simulink model "tank_based_bi_teleop_pf_kalman"  (R2020b)
settings: Solver=FixedStepAuto  StartTime=0.0  StopTime=30  FixedStep=Ts  RelTol=1e-3
values from neighbouring files (symbols this model uses):
  A = 1    [four_channel_bilateral_teleoperation_kalman_params.m]    (also in four_channel_bilateral_teleoperation_params.m; kalman_test.m = [1 Ts Ts^2/2; 0 1 Ts; 0 0 1]; recursive_estimation.m = [1 Ts Ts^2/2; 0 1 Ts; 0 0 1]; scattering_based_bi_teleop_pf_kalman_params.m)
  alpha = 1    [tank_based_bi_teleop_pf_kalman.m]    (also in tank_based_bi_teleop_pf_params.m; tank_based_bi_teleop_pp_kalman.m; tank_based_bi_teleop_pp_params.m)
  Be = 100    [four_channel_bilateral_teleoperation_architecture_params.m]    (also in four_channel_bilateral_teleoperation_kalman_params.m = 0; four_channel_bilateral_teleoperation_params.m = 0; scattering_based_bi_teleop_pf_kalman_params.m = 10; scattering_based_bi_teleop_pf_params.m = 10)
  beta = 0.2    [tank_based_bi_teleop_pf_kalman.m]    (also in tank_based_bi_teleop_pf_params.m; tank_based_bi_teleop_pp_kalman.m; tank_based_bi_teleop_pp_params.m)
  Bh = 70    [four_channel_bilateral_teleoperation_architecture_params.m]    (also in four_channel_bilateral_teleoperation_kalman_params.m; four_channel_bilateral_teleoperation_params.m; scattering_based_bi_teleop_pf_kalman_params.m = 1.5; scattering_based_bi_teleop_pf_params.m = 1.5)
  Bs = 1    [four_channel_bilateral_teleoperation_architecture_params.m]    (also in four_channel_bilateral_teleoperation_kalman_params.m = 3.2; four_channel_bilateral_teleoperation_params.m = 3.2; scattering_based_bi_teleop_pf_kalman_params.m = 40; scattering_based_bi_teleop_pf_params.m = 3)
  delay = 1    [scattering_based_bi_teleop_pf_kalman_params.m]    (also in scattering_based_bi_teleop_pf_params.m; scattering_based_bi_teleop_pp_kalman_params.m; scattering_based_bi_teleop_pp_params.m; tank_based_bi_teleop_pf_kalman.m)
  Dm = 5    [four_channel_bilateral_teleoperation_architecture_params.m]    (also in four_channel_bilateral_teleoperation_kalman_params.m = 0; four_channel_bilateral_teleoperation_params.m = 0; scattering_based_bi_teleop_pf_kalman_params.m = 0; scattering_based_bi_teleop_pf_params.m = 0)
  Ds = 10    [four_channel_bilateral_teleoperation_architecture_params.m]    (also in four_channel_bilateral_teleoperation_kalman_params.m = 0; four_channel_bilateral_teleoperation_params.m = 0; scattering_based_bi_teleop_pf_kalman_params.m = 0; scattering_based_bi_teleop_pf_params.m = 0)
  Fc = 1    [four_channel_bilateral_teleoperation_kalman_params.m]    (also in four_channel_bilateral_teleoperation_params.m; kalman_test.m = 10; scattering_based_bi_teleop_pf_kalman_params.m = 0.1; scattering_based_bi_teleop_pf_params.m)
  Fip = 1    [four_channel_bilateral_teleoperation_kalman_params.m]    (also in four_channel_bilateral_teleoperation_params.m; scattering_based_bi_teleop_pf_kalman_params.m = 5; scattering_based_bi_teleop_pf_params.m; scattering_based_bi_teleop_pp_kalman_params.m = 5)
  h_limit = 1    [tank_based_bi_teleop_pf_kalman.m]    (also in tank_based_bi_teleop_pf_params.m; tank_based_bi_teleop_pp_kalman.m; tank_based_bi_teleop_pp_params.m = 1.5)
  H_master_init = 100    [tank_based_bi_teleop_pf_kalman.m]    (also in tank_based_bi_teleop_pf_params.m; tank_based_bi_teleop_pp_kalman.m = 5; tank_based_bi_teleop_pp_params.m = 1)
  H_slave_init = 100    [tank_based_bi_teleop_pf_kalman.m]    (also in tank_based_bi_teleop_pf_params.m; tank_based_bi_teleop_pp_kalman.m = 5; tank_based_bi_teleop_pp_params.m = 1)
  Ih = 2    [scattering_based_bi_teleop_pf_kalman_params.m]    (also in scattering_based_bi_teleop_pp_kalman_params.m; scattering_based_bi_teleop_pp_params.m; tank_based_bi_teleop_pf_kalman.m; tank_based_bi_teleop_pf_params.m)
  Je = 0    [four_channel_bilateral_teleoperation_architecture_params.m]    (also in four_channel_bilateral_teleoperation_kalman_params.m; four_channel_bilateral_teleoperation_params.m; scattering_based_bi_teleop_pf_kalman_params.m; scattering_based_bi_teleop_pf_params.m)
  Jh = 0.5    [four_channel_bilateral_teleoperation_architecture_params.m]    (also in four_channel_bilateral_teleoperation_kalman_params.m; four_channel_bilateral_teleoperation_params.m; scattering_based_bi_teleop_pf_kalman_params.m = 0; scattering_based_bi_teleop_pf_params.m = 0.05)
  Ke = 200    [four_channel_bilateral_teleoperation_architecture_params.m]    (also in four_channel_bilateral_teleoperation_kalman_params.m = 50; four_channel_bilateral_teleoperation_params.m = 50; scattering_based_bi_teleop_pf_kalman_params.m; scattering_based_bi_teleop_pf_params.m)
  Kh = 2000    [four_channel_bilateral_teleoperation_architecture_params.m]    (also in four_channel_bilateral_teleoperation_kalman_params.m; four_channel_bilateral_teleoperation_params.m; scattering_based_bi_teleop_pf_kalman_params.m = 1; scattering_based_bi_teleop_pf_params.m = 0)
  Ks = 1    [four_channel_bilateral_teleoperation_architecture_params.m]    (also in four_channel_bilateral_teleoperation_kalman_params.m = 4; four_channel_bilateral_teleoperation_params.m = 4; scattering_based_bi_teleop_pf_kalman_params.m = 50; scattering_based_bi_teleop_pf_params.m = 110)
  Mm = 0.5    [four_channel_bilateral_teleoperation_architecture_params.m]    (also in four_channel_bilateral_teleoperation_kalman_params.m; four_channel_bilateral_teleoperation_params.m; scattering_based_bi_teleop_pf_kalman_params.m; scattering_based_bi_teleop_pf_params.m)
  Ms = 2    [four_channel_bilateral_teleoperation_architecture_params.m]    (also in four_channel_bilateral_teleoperation_kalman_params.m; four_channel_bilateral_teleoperation_params.m; scattering_based_bi_teleop_pf_kalman_params.m; scattering_based_bi_teleop_pf_params.m)
  Ph = 2000    [four_channel_bilateral_teleoperation_kalman_params.m]    (also in four_channel_bilateral_teleoperation_params.m = 50500; scattering_based_bi_teleop_pf_kalman_params.m = 5; scattering_based_bi_teleop_pf_params.m = 23; scattering_based_bi_teleop_pp_kalman_params.m = 6)
  Ts = 0.001    [four_channel_bilateral_teleoperation_kalman_params.m]    (also in four_channel_bilateral_teleoperation_params.m; kalman_test.m; recursive_estimation.m; scattering_based_bi_teleop_pf_kalman_params.m)
  VarianceForces = 0.01    [four_channel_bilateral_teleoperation_kalman_params.m]    (also in four_channel_bilateral_teleoperation_params.m; scattering_based_bi_teleop_pf_kalman_params.m; scattering_based_bi_teleop_pp_kalman_params.m; scattering_based_bi_teleop_pp_params.m)
  VarianceVelocities = 0.001    [four_channel_bilateral_teleoperation_kalman_params.m]    (also in four_channel_bilateral_teleoperation_params.m; scattering_based_bi_teleop_pf_kalman_params.m = 1e-05; scattering_based_bi_teleop_pp_kalman_params.m = 1e-05; scattering_based_bi_teleop_pp_params.m = 1e-05)
settings Model: Creator=anuj  LastModifiedBy=filippo

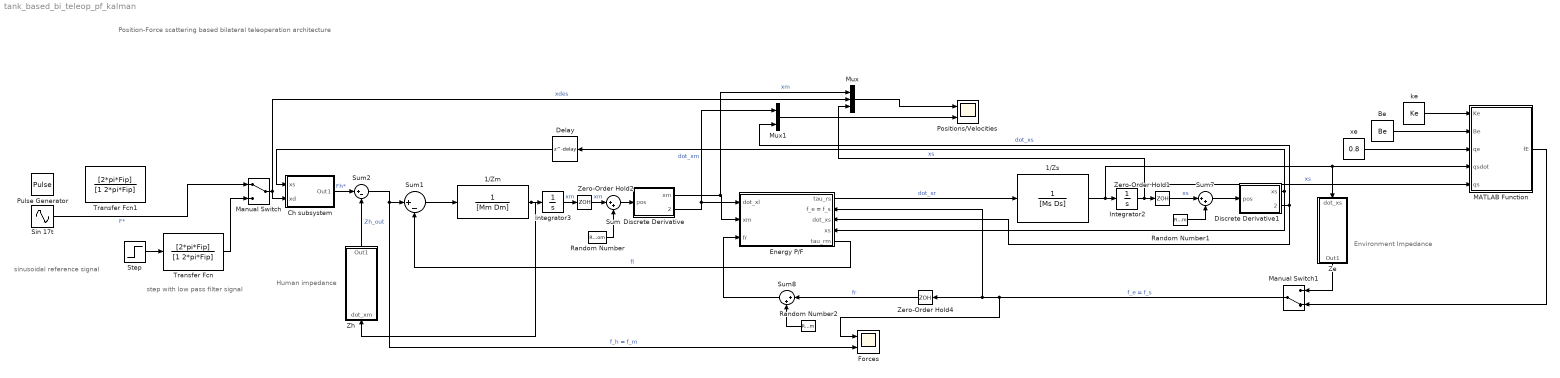
== system tank_based_bi_teleop_pf_kalman ==
  note: Position-Force scattering based bilateral teleoperation architecture
  note: Environment Impedance
  note: Human impedance
  note: sinusoidal reference signal
  note: step with low pass filter signal
  1/Zm : TransferFcn  Denominator=[Mm Dm]
  1/Zs : TransferFcn  Denominator=[Ms Ds]
  Be : Constant  Value=Be
  Ch subsystem : Subsystem
  Delay : Delay  DelayLength=delay  SampleTime=Ts
  Discrete Derivative : Subsystem
  Discrete Derivative1 : Subsystem
  Energy P/F : Subsystem
      settings: PortSchema="{\"entries\":[{\"content\":{\"sides\":[{\"content\":{\"connectorIds\":[\"In1\",\"In2\",\"In3\"]},\"type\":\"ConnectorPlacement.EquallySpacedRectSide\",\"uuid\":\"f2b5b233-4bc9-48fa-8c02-3c8bfabc8edf\"},{\"content\":{\"connectorIds\":[\"Out1\",\"In4\",\"In5\",\"In6\",\"Out2\"],\"side\":\"RIGHT\"},\"type\":\"ConnectorPlacement.EquallySpacedRectSide\",\"uuid\":\"567bdcc6-c695-4210-9521-fb074471be82\"},{\"content\":{\"connectorIds\":[],\"side\":\"TOP\"},\"type\":\"ConnectorPlacement.EquallySpacedRectSide\",\"uuid\":\"1a36b9db-f8a2-44fb-9901-095b7ca2258a\"},{\"content\":{\"connectorIds\":[],\"side\":\"HIDDEN\"},\"type\":\"ConnectorPlacement.EquallySpacedRectSide\",\"uuid\":\"2e8b54c5-18c4-4c1b-a8a4-ee42e67d82c7\"}]},\"type\":\"ConnectorPlacement.EquallySpacedConnector\",\"uuid\":\"569d959e-ea5b-42c6-b188-2deb8683cad8\"}],\"packageUris\":[\"http://schema.mathworks.com/mf0/Connector/R2020b\"],\"version\":\"1.0\"}"
  Forces : Scope  NumInputPorts=2
  Integrator2 : Integrator
  Integrator3 : Integrator
  MATLAB Function : MATLAB Function  TreatAsAtomicUnit=on
  Manual Switch : ManualSwitch
  Manual Switch1 : ManualSwitch  CurrentSetting=0
  Mux : Mux  Inputs=3
  Mux1 : Mux  Inputs=2
  Positions/Velocities : Scope  NumInputPorts=2
  Pulse Generator : DiscretePulseGenerator  PulseType=Time based  Amplitude=A  PulseWidth=50  PhaseDelay=1
  Random Number : RandomNumber  Variance=VarianceVelocities  SampleTime=Ts
  Random Number1 : RandomNumber  Variance=VarianceVelocities  SampleTime=Ts
  Random Number2 : RandomNumber  Variance=VarianceForces  SampleTime=Ts
  Sin 17t : Sin  Amplitude=A  Frequency=2*pi*Fc  SampleTime=0
  Step : Step  After=A  SampleTime=0
  Sum : Sum  Inputs=|++
  Sum1 : Sum  Inputs=|+-
  Sum2 : Sum  Inputs=|+-
  Sum7 : Sum  Inputs=|++
  Sum8 : Sum  Inputs=|++
  Transfer Fcn : TransferFcn  Numerator=[2*pi*Fip]  Denominator=[1 2*pi*Fip]
  Transfer Fcn1 : TransferFcn  Numerator=[2*pi*Fip]  Denominator=[1 2*pi*Fip]
  Ze : Subsystem
  Zero-Order Hold1 : ZeroOrderHold  SampleTime=Ts
  Zero-Order Hold2 : ZeroOrderHold  SampleTime=Ts
  Zero-Order Hold4 : ZeroOrderHold  SampleTime=Ts
  Zh : Subsystem
  ke : Constant  Value=Ke
  xe : Constant  Value=0.8
  wires:
  Sum2/1 -> Forces/2, Sum1/1  "f_h = f_m"
  1/Zm/1 -> Zh/1(dot_xm), Integrator3/1
  Sum1/1 -> 1/Zm/1
  Energy P/F/2(tau_rm) -> Sum1/2  "fl"
  Manual Switch1/1 -> Energy P/F/4(f_e = f_s), Zero-Order Hold4/1, Forces/1  "f_e = f_s"
  Be/1 -> MATLAB Function/2(Be)
  xe/1 -> MATLAB Function/3(qe)
  ke/1 -> MATLAB Function/1(Ke)
  Transfer Fcn/1 -> Manual Switch/2
  Step/1 -> Transfer Fcn/1
  Zh/1(Out1) -> Sum2/2  "Zh_out"
  Discrete Derivative1/2(dot_xs) -> Energy P/F/5(dot_xs), Mux1/2  "dot_xs"
  1/Zs/1 -> Integrator2/1, Ze/1(dot_xs), MATLAB Function/4(qsdot)
  Integrator2/1 -> Zero-Order Hold1/1, Mux/3, MATLAB Function/5(qs)  "xs"
  Zero-Order Hold1/1 -> Sum7/1  "xs"
  Integrator3/1 -> Zero-Order Hold2/1  "xm"
  Discrete Derivative/2(dot_xm) -> Mux1/1, Energy P/F/1(dot_xl)  "dot_xm"
  Ze/1(Out1) -> Manual Switch1/1
  MATLAB Function/1(fE) -> Manual Switch1/2
  Mux1/1 -> Positions/Velocities/2
  Mux/1 -> Positions/Velocities/1
  Manual Switch/1 -> Mux/2, Ch subsystem/2(xd)  "xdes"
  Ch subsystem/1(Out1) -> Sum2/1  "Fh*"
  Energy P/F/1(tau_rs) -> 1/Zs/1  "dot_xr"
  Delay/1 -> Ch subsystem/1(xs)
  Sin 17t/1 -> Manual Switch/1  "F*"
  Sum/1 -> Discrete Derivative/1(pos)
  Random Number/1 -> Sum/2
  Zero-Order Hold2/1 -> Sum/1  "xm"
  Discrete Derivative/1(xm) -> Mux/1, Energy P/F/2(xm)  "xm"
  Random Number2/1 -> Sum8/2
  Zero-Order Hold4/1 -> Sum8/1  "fr"
  Sum8/1 -> Energy P/F/3(fr)
  Random Number1/1 -> Sum7/2
  Sum7/1 -> Discrete Derivative1/1(pos)
  Discrete Derivative1/1(xs) -> Energy P/F/6(xs), Delay/1  "xs"

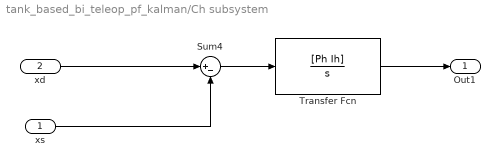
== system tank_based_bi_teleop_pf_kalman/Ch subsystem ==
  xs : Inport
  xd : Inport  Port=2
  Sum4 : Sum  Inputs=|+-
  Transfer Fcn : TransferFcn  Numerator=[Ph Ih]  Denominator=[1 0]
  Out1 : Outport
  wires:
  xd/1 -> Sum4/1
  xs/1 -> Sum4/2
  Sum4/1 -> Transfer Fcn/1
  Transfer Fcn/1 -> Out1/1

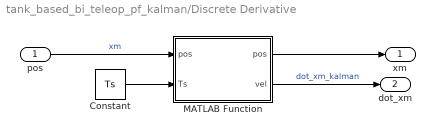
== system tank_based_bi_teleop_pf_kalman/Discrete Derivative ==
  pos : Inport
  Constant : Constant  Value=Ts
  MATLAB Function : MATLAB Function  TreatAsAtomicUnit=on
  xm : Outport
  dot_xm : Outport  Port=2
  wires:
  pos/1 -> MATLAB Function/1("pos ")  "xm"
  Constant/1 -> MATLAB Function/2(Ts)
  MATLAB Function/1(pos) -> xm/1
  MATLAB Function/2(vel) -> dot_xm/1  "dot_xm_kalman"

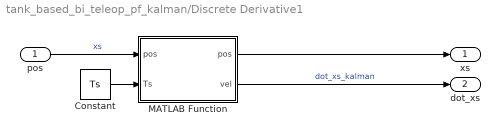
== system tank_based_bi_teleop_pf_kalman/Discrete Derivative1 ==
  pos : Inport
  Constant : Constant  Value=Ts
  MATLAB Function : MATLAB Function  TreatAsAtomicUnit=on
  xs : Outport
  dot_xs : Outport  Port=2
  wires:
  pos/1 -> MATLAB Function/1("pos ")  "xs"
  Constant/1 -> MATLAB Function/2(Ts)
  MATLAB Function/1(pos) -> xs/1
  MATLAB Function/2(vel) -> dot_xs/1  "dot_xs_kalman"

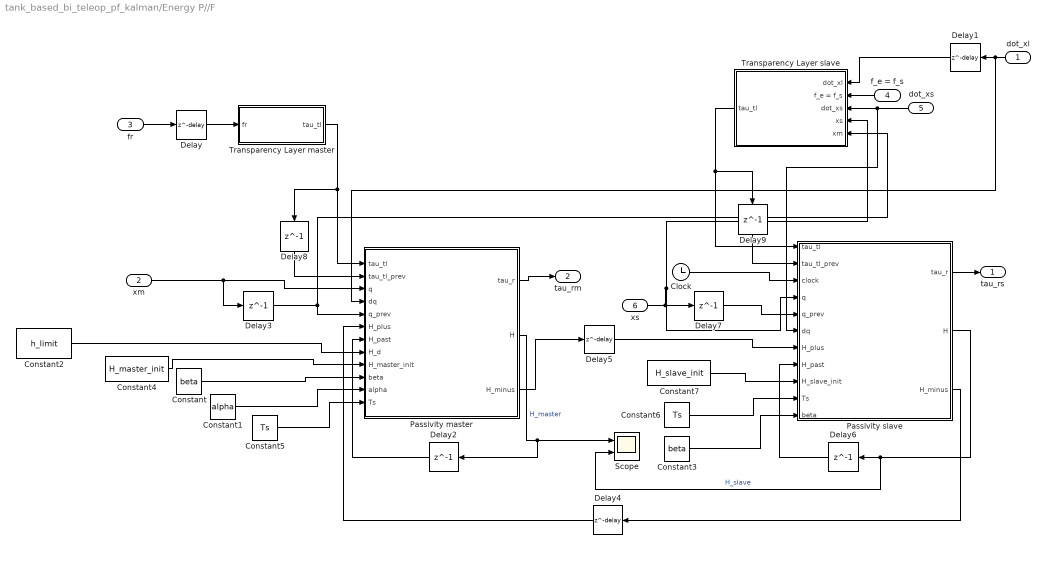
== system tank_based_bi_teleop_pf_kalman/Energy P//F ==
  dot_xl : Inport
  xm : Inport  Port=2
  fr : Inport  Port=3
  f_e = f_s : Inport  Port=4
  dot_xs : Inport  Port=5
  xs : Inport  Port=6
  Clock : Clock
  Constant : Constant  Value=beta
  Constant1 : Constant  Value=alpha
  Constant2 : Constant  Value=h_limit
  Constant3 : Constant  Value=beta
  Constant4 : Constant  Value=H_master_init
  Constant5 : Constant  Value=Ts
  Constant6 : Constant  Value=Ts
  Constant7 : Constant  Value=H_slave_init
  Delay{,1,4..5} (4 alike) : Delay  DelayLength=delay  SampleTime=Ts
  Delay{2..3,6..9} (6 alike) : Delay  DelayLength=1  SampleTime=Ts
  Passivity master : MATLAB Function  TreatAsAtomicUnit=on
  Passivity slave : MATLAB Function  TreatAsAtomicUnit=on
  Scope : Scope  NumInputPorts=2
  Transparency Layer master : Subsystem
  Transparency Layer slave : Subsystem
  tau_rs : Outport
  tau_rm : Outport  Port=2
  wires:
  dot_xl/1 -> Passivity master/4(dq), Delay1/1
  fr/1 -> Delay/1
  Delay2/1 -> Passivity master/7(H_past)
  xm/1 -> Passivity master/3(q), Delay3/1
  Delay3/1 -> Transparency Layer slave/5(xm), Passivity master/5(q_prev)
  Passivity slave/2(H) -> Scope/2, Delay6/1  "H_slave"
  Delay4/1 -> Passivity master/6(H_plus)
  Passivity master/3(H_minus) -> Delay5/1
  Delay5/1 -> Passivity slave/7(H_plus)
  xs/1 -> Transparency Layer slave/4(xs), Passivity slave/4(q), Delay7/1
  Delay6/1 -> Passivity slave/8(H_past)
  Delay7/1 -> Passivity slave/5(q_prev)
  Constant/1 -> Passivity master/10(beta)
  Constant1/1 -> Passivity master/11(alpha)
  Constant2/1 -> Passivity master/8(H_d)
  Passivity master/2(H) -> Delay2/1, Scope/1  "H_master"
  Passivity slave/3(H_minus) -> Delay4/1
  Constant3/1 -> Passivity slave/11(beta)
  Constant4/1 -> Passivity master/9(H_master_init)
  Constant5/1 -> Passivity master/12(Ts)
  Constant6/1 -> Passivity slave/10(Ts)
  Constant7/1 -> Passivity slave/9(H_slave_init)
  Clock/1 -> Passivity slave/3(clock)
  Delay/1 -> Transparency Layer master/1(fr)
  Transparency Layer master/1(tau_tl) -> Delay8/1, Passivity master/1(tau_tl)
  f_e = f_s/1 -> Transparency Layer slave/2(f_e = f_s)
  dot_xs/1 -> Passivity slave/6(dq), Transparency Layer slave/3(dot_xs)
  Delay1/1 -> Transparency Layer slave/1(dot_xl)
  Transparency Layer slave/1(tau_tl) -> Delay9/1, Passivity slave/1(tau_tl)
  Passivity master/1(tau_r) -> tau_rm/1
  Passivity slave/1(tau_r) -> tau_rs/1
  Delay8/1 -> Passivity master/2(tau_tl_prev)
  Delay9/1 -> Passivity slave/2(tau_tl_prev)

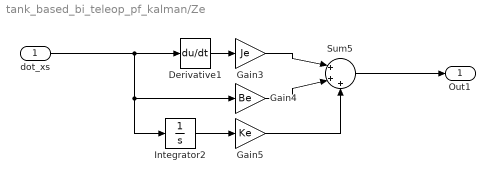
== system tank_based_bi_teleop_pf_kalman/Ze ==
  dot_xs : Inport
  Derivative1 : Derivative
  Gain3 : Gain  Gain=Je
  Gain4 : Gain  Gain=Be
  Gain5 : Gain  Gain=Ke
  Integrator2 : Integrator
  Sum5 : Sum  Inputs=|+++
  Out1 : Outport
  wires:
  Gain4/1 -> Sum5/2
  Gain3/1 -> Sum5/1
  Gain5/1 -> Sum5/3
  Sum5/1 -> Out1/1
  Integrator2/1 -> Gain5/1
  dot_xs/1 -> Integrator2/1, Gain4/1, Derivative1/1
  Derivative1/1 -> Gain3/1

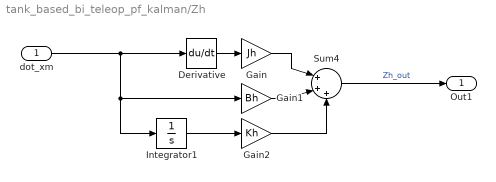
== system tank_based_bi_teleop_pf_kalman/Zh ==
  dot_xm : Inport
  Derivative : Derivative
  Gain : Gain  Gain=Jh
  Gain1 : Gain  Gain=Bh
  Gain2 : Gain  Gain=Kh
  Integrator1 : Integrator
  Sum4 : Sum  Inputs=|+++
  Out1 : Outport
  wires:
  Derivative/1 -> Gain/1
  Integrator1/1 -> Gain2/1
  Gain2/1 -> Sum4/3
  Gain1/1 -> Sum4/2
  Gain/1 -> Sum4/1
  Sum4/1 -> Out1/1  "Zh_out"
  dot_xm/1 -> Gain1/1, Integrator1/1, Derivative/1

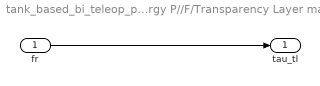
== system tank_based_bi_teleop_pf_kalman/Energy P//F/Transparency Layer master ==
  fr : Inport
  tau_tl : Outport
  wires:
  fr/1 -> tau_tl/1

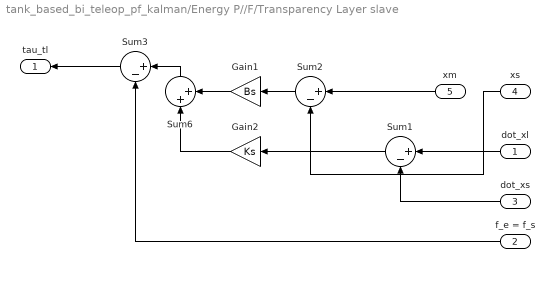
== system tank_based_bi_teleop_pf_kalman/Energy P//F/Transparency Layer slave ==
  dot_xl : Inport
  f_e = f_s : Inport  Port=2
  dot_xs : Inport  Port=3
  xs : Inport  Port=4
  xm : Inport  Port=5
  Gain1 : Gain  Gain=Bs
  Gain2 : Gain  Gain=Ks
  Sum1 : Sum  Inputs=|+-
  Sum2 : Sum  Inputs=|+-
  Sum3 : Sum  Inputs=|+-
  Sum6 : Sum  Inputs=|++
  tau_tl : Outport
  wires:
  Sum6/1 -> Sum3/1
  Sum1/1 -> Gain2/1
  Sum3/1 -> tau_tl/1
  dot_xs/1 -> Sum1/2
  Sum2/1 -> Gain1/1
  dot_xl/1 -> Sum1/1
  f_e = f_s/1 -> Sum3/2
  Gain2/1 -> Sum6/1
  Gain1/1 -> Sum6/2
  xm/1 -> Sum2/1
  xs/1 -> Sum2/2

== matlab function tank_based_bi_teleop_pf_kalman/Energy P//F/Passivity master ==
  data: tau_tl input; tau_tl_prev input; tau_r output; q input; dq input; q_prev input; H_plus input; H_past input; H_d input; H_master_init input; beta input; alpha input; H output; H_minus output; Ts input
function [tau_r,H,H_minus] = passivity_master(tau_tl, tau_tl_prev, q, dq, q_prev, H_plus, H_past, H_d, H_master_init, beta, alpha, Ts)
    persistent init
    if isempty(init)
        init = 0;
        H_past = H_master_init;
    end
    deltaH = tau_tl_prev*(q-q_prev);
    
    H = H_past + H_plus - deltaH;
    
    tau_max = abs(tau_tl);
    if H <= 0
        tau_max = 0;
    end
    
    if abs(dq) > 0.001
        tau_max = min(tau_max, abs(H/(dq*Ts)));
    end
    
    tau_pl = sign(tau_tl)*min(abs(tau_tl),tau_max);
    
    % TLC action to get energy from user
    if (H_d > H)
        tau_tlc = -alpha*(H_d-H)*dq;
    else
        tau_tlc = 0;
    end
    
    % Send fixed fraction of energy
    H_minus = beta*H;
    H = H - H_minus;
    
    tau_r = tau_pl + tau_tlc;
end

== matlab function tank_based_bi_teleop_pf_kalman/MATLAB Function ==
  data: Ke input; fE output; Be input; qe input; qsdot input; qs input
function fE = environment(Ke, Be, qe, qsdot, qs)
    if qs > qe
        fE = Ke * (qs - qe) + Be * qsdot; % Plot both contributions Ke and Be
    else
        fE = 0;
    end
end

== matlab function tank_based_bi_teleop_pf_kalman/Energy P//F/Passivity slave ==
  data: tau_tl input; tau_tl_prev input; clock input; tau_r output; q input; q_prev input; dq input; H_plus input; H_past input; H_slave_init input; Ts input; H output; H_minus output; beta input
function [tau_r, H, H_minus] = passivity_slave(tau_tl, tau_tl_prev, clock, q, q_prev, dq, H_plus, H_past,H_slave_init,Ts, beta)
    if clock == 0
        H_past = H_slave_init;
    end
    deltaH = tau_tl_prev*(q-q_prev);
    H = H_past + H_plus - deltaH;
    
    tau_max = abs(tau_tl);
    if H <= 0
        tau_max = 0;
    end
    
    if abs(dq) > 0.001
        tau_max = min(tau_max, abs(H/(dq*Ts)));
    end
     
    tau_r = sign(tau_tl)*min(abs(tau_tl),tau_max);
    
    % Send fixed fraction of energy
    H_minus = beta*H;
    H = H - H_minus;
end

== matlab function tank_based_bi_teleop_pf_kalman/Discrete Derivative/MATLAB Function ==
  data: pos output; pos input; vel output; Ts input
function [pos, vel] = kalman(pos, Ts)
    persistent P A C Q R x_filter_old P_filter_old
    if isempty(P)
        P = 0;
        x_filter_old=[pos; 0];
        P_filter_old=0.1*eye(2);
        A=[1 Ts; 0 1];
        C=[1 0];
        q=1000000;
        Q=q*[Ts^2/2;Ts]*[Ts^2/2;Ts]';
        R=1;
    end

    % Prediction step (A priori estimation)
    x_kplus1_k = A*x_filter_old;
    P_kplus1_k = A*P_filter_old*A'+Q;

    % Compute the kalman gain
    K = P_kplus1_k * C' * inv(C * P_kplus1_k * C' + R);

    % Calculate the estimation step
    x_kplus1_kplus1 = x_kplus1_k + K *(pos - C * x_kplus1_k);
    P_kplus1_kplus1 = P_kplus1_k - P_kplus1_k * C' * inv(C * P_kplus1_k * C' + R) * C * P_kplus1_k;
    
    % Next step iteration
    x_filter_old = x_kplus1_kplus1;
    P_filter_old = P_kplus1_kplus1;
    
    pos = x_kplus1_kplus1(1,:);
    vel = x_kplus1_kplus1(2,:);
end

== matlab function tank_based_bi_teleop_pf_kalman/Discrete Derivative1/MATLAB Function ==
  data: pos output; pos input; vel output; Ts input
function [pos, vel] = kalman(pos, Ts)
    persistent P A C Q R x_filter_old P_filter_old
    if isempty(P)
        P = 0;
        x_filter_old=[pos; 0];
        P_filter_old=0.1*eye(2);
        A=[1 Ts; 0 1];
        C=[1 0];
        q=1000000;
        Q=q*[Ts^2/2;Ts]*[Ts^2/2;Ts]';
        R=1;
    end

    % Prediction step (A priori estimation)
    x_kplus1_k = A*x_filter_old;
    P_kplus1_k = A*P_filter_old*A'+Q;

    % Compute the kalman gain
    K = P_kplus1_k * C' * inv(C * P_kplus1_k * C' + R);

    % Calculate the estimation step
    x_kplus1_kplus1 = x_kplus1_k + K *(pos - C * x_kplus1_k);
    P_kplus1_kplus1 = P_kplus1_k - P_kplus1_k * C' * inv(C * P_kplus1_k * C' + R) * C * P_kplus1_k;
    
    % Next step iteration
    x_filter_old = x_kplus1_kplus1;
    P_filter_old = P_kplus1_kplus1;
    
    pos = x_kplus1_kplus1(1,:);
    vel = x_kplus1_kplus1(2,:);
end
